simulink model "muxbus"  (R2022b)
settings: Solver=VariableStepAuto  StartTime=0.0  StopTime=10.0  RelTol=1e-3
InitFcn:
  | x=23;
  | y=45;
  | z=90;
model workspace (MAT data in the model file):
  x = 4
  y = 5
  z = 6
settings Model: ParameterArgumentNames=x  Creator=Brigosha_Guest  LastModifiedBy=Brigosha_Guest
settings ConfigComp: CovMetricSettings=dcmwe

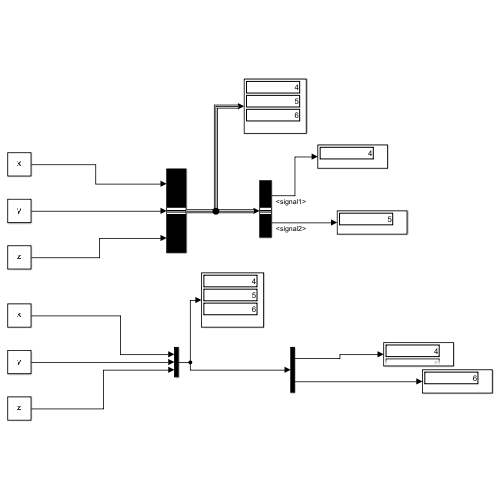
[thumbnail: Simulink's stored preview of the top-level diagram]
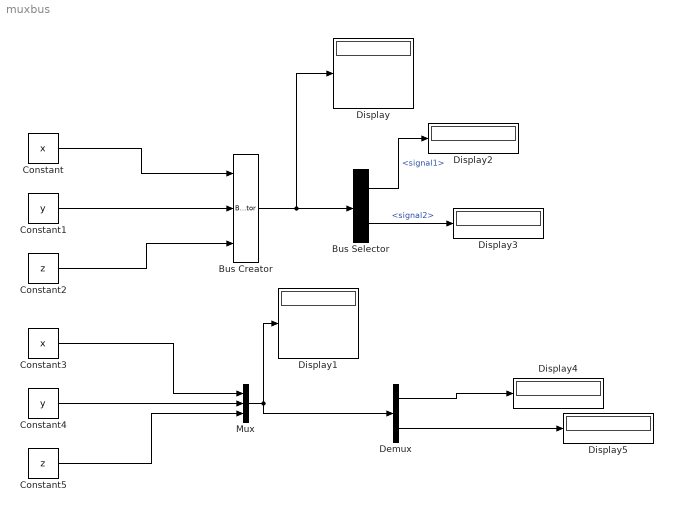
== system muxbus ==
  Bus Creator : BusCreator  Inputs=3
  Bus Selector : BusSelector  OutputSignals=signal1,signal2
  Constant : Constant  Value=x
  Constant1 : Constant  Value=y
  Constant2 : Constant  Value=z
  Constant3 : Constant  Value=x
  Constant4 : Constant  Value=y
  Constant5 : Constant  Value=z
  Demux : Demux  Outputs=2
  Display{,1..5} (6 alike) : Display
  Mux : Mux  Inputs=3
  wires:
  Constant/1 -> Bus Creator/1
  Constant1/1 -> Bus Creator/2
  Constant2/1 -> Bus Creator/3
  Bus Creator/1 -> Bus Selector/1, Display/1
  Mux/1 -> Demux/1, Display1/1
  Constant5/1 -> Mux/3
  Constant4/1 -> Mux/2
  Constant3/1 -> Mux/1
  Bus Selector/1 -> Display2/1  "<signal1>"
  Bus Selector/2 -> Display3/1  "<signal2>"
  Demux/1 -> Display4/1
  Demux/2 -> Display5/1
